simulink model "interleaver"  (R2022b)
settings: Solver=VariableStepAuto  StartTime=0.0  StopTime=10  RelTol=1e-3
libraries: commblkintrlv2 x2
settings Model: Creator=senolgulgonul  LastModifiedBy=senol
settings SolverCC: AlgebraicLoopSolver=TrustRegion
settings DataIOCC: ReturnWorkspaceOutputs=off
settings DebuggingCC: UnconnectedInputMsg=warning  UnconnectedOutputMsg=warning  UnconnectedLineMsg=warning  SFMachineParentedDataDiag=warning  ArithmeticOperatorsInVariantConditions=warning
settings ModelReferenceCC: EnableRefExpFcnMdlSchedulingChecks=on
settings SFSimCC: SimUseLocalCustomCode=off  CustomCodeUndefinedFunction=UseInterfaceOnly
settings RTWCC: RTWUseLocalCustomCode=off
settings CodeAppCC: StateflowObjectComments=on

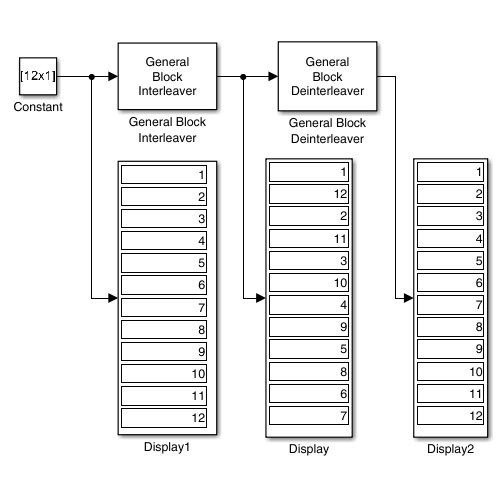
[thumbnail: Simulink's stored preview of the top-level diagram]
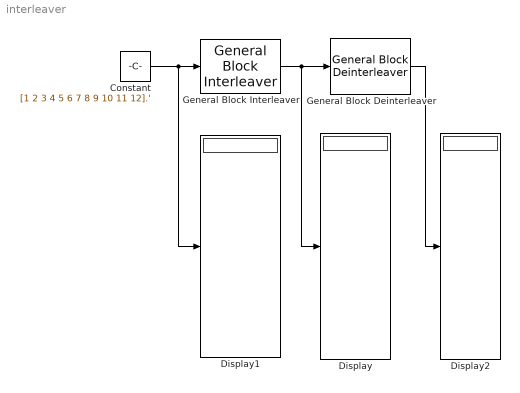
== system interleaver ==
  Constant : Constant  Value=[1 2 3 4 5 6 7 8 9 10 11 12].'  SampleTime=1
  Display : Display
  Display1 : Display
  Display2 : Display
  General Block Deinterleaver : commblkintrlv2/General Block Deinterleaver  StatePerturbationForJacobian=1.0e-05  permutationVectorSource=Dialog  elements="[ 1 12 2 11 3 10 4 9 5 8 6 7  ]'"
  General Block Interleaver : commblkintrlv2/General Block Interleaver  StatePerturbationForJacobian=1.0e-05  permutationVectorSource=Dialog  elements="[ 1 12 2 11 3 10 4 9 5 8 6 7  ]'"
  wires:
  General Block Interleaver/1 -> General Block Deinterleaver/1, Display/1
  Constant/1 -> General Block Interleaver/1, Display1/1
  General Block Deinterleaver/1 -> Display2/1
